simulink model "pure_pursuit"  (R2025b)
settings: Solver=ode45  StartTime=0.0  StopTime=inf  RelTol=1e-3
model workspace (MAT data in the model file):
  SL_ROS_VariableLengthArrays_MaxSizes.CommonInfo.ArrayTruncateAction = 'EmitWarning'
  SL_ROS_VariableLengthArrays_MaxSizes.MsgTypeMap = containers.Map
  SL_ROS_VariableLengthArrays_MaxSizes.MsgTypeMap.serialization.keys = {'autoware_planning_msgs/Path'}
  SL_ROS_VariableLengthArrays_MaxSizes.MsgTypeMap.serialization.values{1}(1).PropertyName = 'left_bound'
  SL_ROS_VariableLengthArrays_MaxSizes.MsgTypeMap.serialization.values{1}(1).DataType = 'geometry_msgs/Point'
  SL_ROS_VariableLengthArrays_MaxSizes.MsgTypeMap.serialization.values{1}(1).MaxLength = 159
  SL_ROS_VariableLengthArrays_MaxSizes.MsgTypeMap.serialization.values{1}(2).PropertyName = 'points'
  SL_ROS_VariableLengthArrays_MaxSizes.MsgTypeMap.serialization.values{1}(2).DataType = 'autoware_planning_msgs/PathPoint'
  SL_ROS_VariableLengthArrays_MaxSizes.MsgTypeMap.serialization.values{1}(2).MaxLength = 159
  SL_ROS_VariableLengthArrays_MaxSizes.MsgTypeMap.serialization.values{1}(3).PropertyName = 'right_bound'
  SL_ROS_VariableLengthArrays_MaxSizes.MsgTypeMap.serialization.values{1}(3).DataType = 'geometry_msgs/Point'
  SL_ROS_VariableLengthArrays_MaxSizes.MsgTypeMap.serialization.values{1}(3).MaxLength = 159
  SL_ROS_VariableLengthArrays_MaxSizes.MsgTypeMap.serialization.uniformity = 0
  SL_ROS_VariableLengthArrays_MaxSizes.MsgTypeMap.serialization.keyType = 'char'
  SL_ROS_VariableLengthArrays_MaxSizes.MsgTypeMap.serialization.valueType = 'any'
values from neighbouring files (symbols this model uses):
  L = 3    [autoware_referance_path_creater.m]    (also in pure_pursuit_parameters.m)
  ld = 5    [autoware_referance_path_creater.m]    (also in pure_pursuit_parameters.m = 3)
  max_ld = 10    [autoware_referance_path_creater.m]    (also in pure_pursuit_parameters.m)
  max_steer_cmd = 0.5    [autoware_referance_path_creater.m]    (also in pure_pursuit_parameters.m)
  max_vel = 10    [autoware_referance_path_creater.m]    (also in pure_pursuit_parameters.m)
  min_ld = 3    [autoware_referance_path_creater.m]    (also in pure_pursuit_parameters.m)
  min_steer_cmd = 0.0    (= 0)    [autoware_referance_path_creater.m]    (also in pure_pursuit_parameters.m)
  min_vel = 5    [autoware_referance_path_creater.m]    (also in pure_pursuit_parameters.m)
  psi_o = atan2(dy0, dx0)    [autoware_referance_path_creater.m]    (also in pure_pursuit_parameters.m = 0)
  x_mean = x_mean(:)    [load_onnx_params.m]    (also in scaler_params.mat = [28.1934460749 74.6575043237 -0.0407059238974])
  X_o = refPose(1,1)    [autoware_referance_path_creater.m]    (also in pure_pursuit_parameters.m)
  x_std = x_std(:)    [load_onnx_params.m]    (also in scaler_params.mat = [17.0789640418 18.417349091 0.180735882078])
  xRef = refPose(:,1)    [autoware_referance_path_creater.m]    (also in pure_pursuit_parameters.m)
  y_mean = y_mean(:)    [load_onnx_params.m]    (also in scaler_params.mat = [7.96333555037 8.54523967985])
  Y_o = refPose(1,2)    [autoware_referance_path_creater.m]    (also in pure_pursuit_parameters.m)
  y_std = y_std(:)    [load_onnx_params.m]    (also in scaler_params.mat = [1.60598708046 1.14713361971])
  yRef = refPose(:,2)    [autoware_referance_path_creater.m]    (also in pure_pursuit_parameters.m)
libraries: autolibshared x6, robotalgslib x5, robotmobilelib x2, pycoexlib x1, ros2lib x1
settings Model: Creator=omer  LastModifiedBy=omer
settings OptimizationCC: DefaultParameterBehavior=Inlined  EnhancedBackFolding=on  PassReuseOutputArgsAs=Individual arguments  ZeroExternalMemoryAtStartup=off  ZeroInternalMemoryAtStartup=off  MaxStackSize=64  OptimizeBlockOrder=speed  DifferentSizesBufferReuse=on  OptimizationCustomize=off  EfficientTunableParamExpr=on
settings DebuggingCC: AlgebraicLoopMsg=none  ParameterTunabilityLossMsg=error
settings HardwareCC: ProdBitPerLong=64.0  ProdHWDeviceType=Intel->x86-64 (Linux 64)
settings SFSimCC: MATLABDynamicMemAlloc=off
settings RTWCC: SystemTargetFile=ert.tlc  HardwareBoard=Robot Operating System 2 (ROS 2)  TLCOptions="-aInlineSetEventsForThisBaseRateFcn=TLC_FALSE -aSuppressMultiTaskScheduler=TLC_FALSE  -aRateBasedStepFcn=0"  TemplateMakefile=ert_default_tmf  Toolchain=Colcon Tools  TargetLang=C++  Description=Embedded Coder
settings CodeAppCC: ForceParamTrailComments=on  IgnoreCustomStorageClasses=off  OperatorAnnotations=on  SimulinkDataObjDesc=on  SFDataObjDesc=on  InsertBlockDesc=on
settings ERTTargetCC: ExtModeTransport=2.0  ExtModeStaticAlloc=on  ExtModeAutomaticAllocSize=off  ExtModeMexFile=ext_xcp  ExtModeIntrfLevel=Level2 - Open  RootIOFormat=Structure reference  CodeInterfacePackaging=C++ class

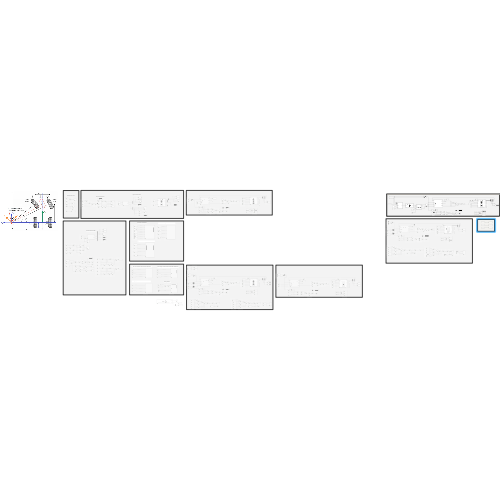
[thumbnail: Simulink's stored preview of the top-level diagram]
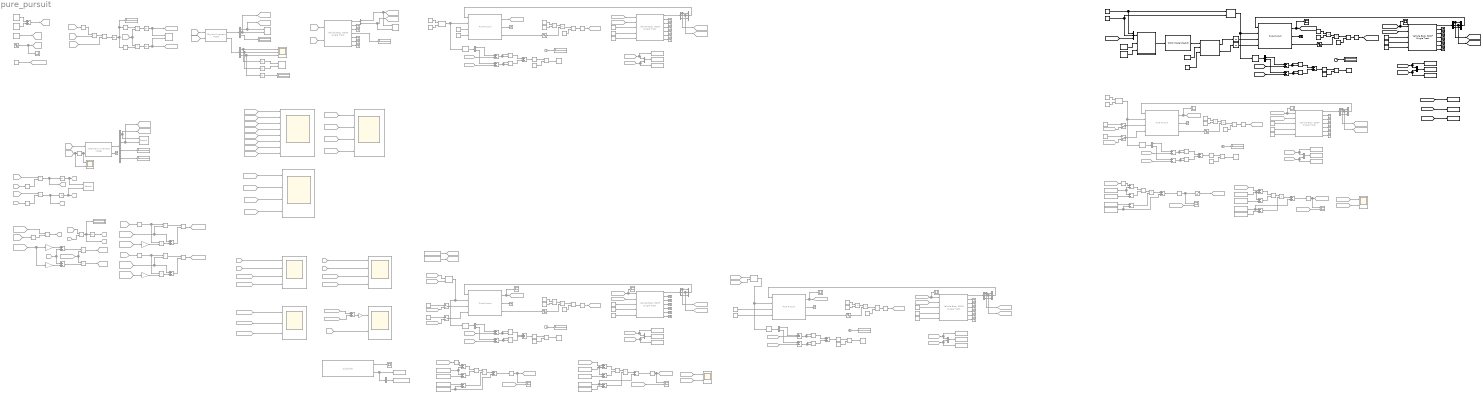
== system pure_pursuit ==
  note: Bicycle Kinematics Model
  note: Bicycle Kinematics Model
  note: Ackerman Kinematics Model
  note: Kinematics Model Inputs
  note: All Kinematics Model Results
  note: Built in and custom Bicycle Kinematics Model Results
  note: Bicycle and Ackerman Kinematics Model Results
  note: Built-in and custom Ackermann Kinematics Model Results
  note: Custom Bicycle and custom Ackermann Kinematics Model Results
  note: Velocity Calculation
  note: Steering Angle Calculation
  Abs{,1..5} (6 alike) : Abs  Commented=on  SaturateOnIntegerOverflow=off
  Ackermann Kinematic Model : robotmobilelib/Ackermann Kinematic Model  Commented=on  WheelBase=3  VehicleSpeedRange=[-10 10]  MaxSteeringAngle=pi/4  InitialState=[0; 0; 0; 0]  SimulateUsing=Interpreted execution
  Add{,1..5,8,11,19,23,32,34} (12 alike) : Sum  Commented=on
  Add{6..7,9..10,12,15..16,22,24,27..28,33,35..36} (14 alike) : Sum  Commented=on  Inputs=+-
  Add{13..14,17..18,25..26,29,31} (8 alike) : Sum  Commented=on  Inputs=-+
  Add37 : Sum  Inputs=+-
  Add38 : Sum
  Add39 : Sum  Inputs=+-
  Angular Velocity : Sin  Commented=on  Amplitude=0.6  Frequency=0.2  SampleTime=0
  Atan{,1,3..4} (4 alike) : Trigonometry  Commented=on  Operator=atan
  Atan5 : Trigonometry  Operator=atan
  Bicycle Kinematic Model : robotmobilelib/Bicycle Kinematic Model  Commented=on  VehicleInputs=Vehicle Speed & Steering Angle  WheelBase=3  VehicleSpeedRange=[-10 10]  MaxSteeringAngle=pi/4  InitialState=[0; 0; 0]  SimulateUsing=Interpreted execution
  Bus Selector{,2,5..6} (4 alike) : BusSelector  Commented=on  OutputSignals=InertFrm.Cg.Disp.X,InertFrm.Cg.Disp.Y,InertFrm.Cg.Ang.psi
  Bus Selector1 : BusSelector  Commented=on  OutputSignals=InertFrm.Cg.Disp.X,InertFrm.Cg.Disp.Y
  Bus Selector4 : BusSelector  Commented=on  OutputSignals=points
  Bus Selector7 : BusSelector  OutputSignals=InertFrm.Cg.Disp.X,InertFrm.Cg.Disp.Y,InertFrm.Cg.Ang.psi
  Clock{,1,3..4} (4 alike) : Clock  Commented=on
  Clock5 : Clock
  Constant : Constant  Commented=on  Value=2.5
  Constant{1,10,42,57} (4 alike) : Constant  Commented=on  Value=2
  Constant{8,11,13,21,43,51,58,70} (8 alike) : Constant  Commented=on  Value=ld
  Constant12 : Constant  Commented=on
  Constant14 : Constant  Commented=on  Value=0.5
  Constant{2,15,45,64} (4 alike) : Constant  Commented=on  Value=X_o
  Constant{3,16,46,65} (4 alike) : Constant  Commented=on  Value=Y_o
  Constant{4,17,47,66} (4 alike) : Constant  Commented=on  Value=psi_o
  Constant18 : Constant  Commented=on  Value=xRef
  Constant19 : Constant  Commented=on  Value=yRef
  Constant20 : Constant  Commented=on  Value=10
  Constant{9,22,52,71} (4 alike) : Constant  Commented=on  Value=L
  Constant23 : Constant  Commented=on  Value=min_steer_cmd
  Constant24 : Constant  Commented=on  Value=max_steer_cmd
  Constant{25,29,55,59} (4 alike) : Constant  Commented=on  Value=min_ld
  Constant{26,30,56,60} (4 alike) : Constant  Commented=on  Value=max_ld
  Constant31 : Constant  Commented=on  Value=min_vel
  Constant32 : Constant  Commented=on  Value=max_vel
  Constant44 : Constant  Commented=on
  Constant48 : Constant  Commented=on  Value=xRef
  Constant49 : Constant  Commented=on  Value=yRef
  Constant5 : Constant  Commented=on  Value=xRef
  Constant50 : Constant  Commented=on  Value=5
  Constant53 : Constant  Commented=on  Value=min_steer_cmd
  Constant54 : Constant  Commented=on  Value=max_steer_cmd
  Constant6 : Constant  Commented=on  Value=yRef
  Constant61 : Constant  Commented=on  Value=min_vel
  Constant62 : Constant  Commented=on  Value=max_vel
  Constant63 : Constant  Commented=on
  Constant67 : Constant  Value=2
  Constant68 : Constant  Value=ld
  Constant69 : Constant  Commented=on  Value=10
  Constant7 : Constant  Commented=on  Value=10
  Constant72 : Constant  Value=0.5
  Constant73 : Constant  Value=X_o
  Constant74 : Constant  Value=Y_o
  Constant75 : Constant  Value=psi_o
  Constant76 : Constant  Value=xRef
  Constant77 : Constant  Value=yRef
  Constant78 : Constant  Value=x_mean
  Constant79 : Constant  Value=x_std
  Constant80 : Constant  Value=L
  Constant81 : Constant  Value=y_mean
  Constant82 : Constant  Value=y_std
  Cos : Trigonometry  Commented=on  Operator=cos
  Cos1 : Trigonometry  Commented=on  Operator=cos
  Cos2 : Trigonometry  Commented=on
  Demux : Demux  Commented=on  Outputs=3
  Demux1 : Demux  Commented=on  Outputs=3
  Demux2 : Demux  Commented=on
  Demux{3..4,6..7} (4 alike) : Demux  Commented=on  Outputs=2
  Demux8 : Demux  Outputs=2
  Derivative : Derivative  Commented=on
  Display{,1..8,10..11} (11 alike) : Display  Commented=on
  Display12 : Display
  Divide{,1..8,10..13} (13 alike) : Product  Commented=on  Inputs=*/
  Divide14 : Product  Inputs=*/
  Dot Product{,1..3,6..9} (8 alike) : DotProduct  Commented=on  OutDataTypeStr=Inherit: Inherit via internal rule
  Dot Product10 : DotProduct  OutDataTypeStr=Inherit: Inherit via internal rule
  Dot Product11 : DotProduct  OutDataTypeStr=Inherit: Inherit via internal rule
  From{,2,5,7..8,37,43,45,56} (9 alike) : From  Commented=on  GotoTag=LinVel
  From{1,3,6,9,38,48,51,57} (8 alike) : From  Commented=on  GotoTag=SteerAngle
  From10 : From  Commented=on  GotoTag=bicycle_block_x
  From11 : From  Commented=on  GotoTag=bicycle_block_y
  From12 : From  Commented=on  GotoTag=bicycle_sub_x
  From13 : From  Commented=on  GotoTag=bicycle_sub_y
  From14 : From  Commented=on  GotoTag=ackerman_block_x
  From15 : From  Commented=on  GotoTag=ackerman_block_y
  From16 : From  Commented=on  GotoTag=bicycle_vel_x
  From17 : From  Commented=on  GotoTag=bicycle_vel_y
  From18 : From  Commented=on  GotoTag=bicycle_block_x
  From19 : From  Commented=on  GotoTag=bicycle_block_y
  From20 : From  Commented=on  GotoTag=bicycle_sub_x
  From21 : From  Commented=on  GotoTag=bicycle_sub_y
  From22 : From  Commented=on  GotoTag=bicycle_block_x
  From23 : From  Commented=on  GotoTag=bicycle_block_y
  From24 : From  Commented=on  GotoTag=ackerman_block_x
  From25 : From  Commented=on  GotoTag=ackerman_block_y
  From26 : From  Commented=on  GotoTag=x
  From27 : From  Commented=on  GotoTag=x_feedback
  From28 : From  Commented=on  GotoTag=y_feedback
  From29 : From  Commented=on  GotoTag=calculated_lin_vel
  From30 : From  Commented=on  GotoTag=y
  From31 : From  Commented=on  GotoTag=ackerman_block_x
  From32 : From  Commented=on  GotoTag=ackerman_block_y
  From33 : From  Commented=on  GotoTag=x
  From34 : From  Commented=on  GotoTag=y
  From35 : From  Commented=on  GotoTag=bicycle_sub_x
  From36 : From  Commented=on  GotoTag=bicycle_sub_y
  From{4,39,49,52} (4 alike) : From  Commented=on  GotoTag=WheelBase
  From40 : From  Commented=on  GotoTag=WheelSeparation
  From41 : From  Commented=on  GotoTag=R
  From42 : From  Commented=on  GotoTag=R
  From44 : From  Commented=on  GotoTag=q
  From46 : From  Commented=on  GotoTag=q
  From47 : From  Commented=on  GotoTag=q_dot
  From50 : From  Commented=on  GotoTag=WheelSeparation
  From53 : From  Commented=on  GotoTag=WheelSeparation
  From54 : From  Commented=on  GotoTag=v_inner_wheel
  From55 : From  Commented=on  GotoTag=v_outer_wheel
  From58 : From  Commented=on  GotoTag=InnerSteeringAngle
  From59 : From  Commented=on  GotoTag=OutterSteeringAngle
  From{60,64..65,69..70,80..81,85..86} (9 alike) : From  Commented=on  GotoTag=steering_cmd
  From61 : From  Commented=on  GotoTag=x_feedback
  From62 : From  Commented=on  GotoTag=y_feedback
  From63 : From  Commented=on  GotoTag=calculated_lin_vel
  From{66..67,77,82..83,91} (6 alike) : From  Commented=on  GotoTag=regulated_ld
  From{68,78,84,92} (4 alike) : From  Commented=on  GotoTag=regulated_vel
  From75 : From  Commented=on  GotoTag=x_feedback
  From76 : From  Commented=on  GotoTag=y_feedback
  From79 : From  Commented=on  GotoTag=calculated_lin_vel
  From87 : From  Commented=on  GotoTag=x_feedback2
  From88 : From  Commented=on  GotoTag=y_feedback2
  From89 : From  Commented=on  GotoTag=calculated_lin_vel2
  From90 : From  Commented=on  GotoTag=steering_cmd2
  From93 : From  Commented=on  GotoTag=test_path_x
  From94 : From  Commented=on  GotoTag=test_path_y
  From95 : From  Commented=on  GotoTag=test_path_x
  From96 : From  Commented=on  GotoTag=test_path_y
  Gain : Gain  Commented=on  Gain=-0.5
  Gain1 : Gain  Commented=on  Gain=0.5
  Gain2 : Gain  Commented=on  Gain=-0.5
  Gain3 : Gain  Commented=on  Gain=0.5
  Gain4 : Gain  Commented=on  Gain=0.5
  Goto : Goto  Commented=on  GotoTag=LinVel
  Goto1 : Goto  Commented=on  GotoTag=SteerAngle
  Goto10 : Goto  Commented=on  GotoTag=bicycle_vel_y
  Goto11 : Goto  Commented=on  GotoTag=WheelSeparation
  Goto12 : Goto  Commented=on  GotoTag=calculated_lin_vel
  Goto13 : Goto  Commented=on  GotoTag=steering_cmd
  Goto14 : Goto  Commented=on  GotoTag=x
  Goto15 : Goto  Commented=on  GotoTag=y
  Goto16 : Goto  Commented=on  GotoTag=R
  Goto17 : Goto  Commented=on  GotoTag=q_dot
  Goto18 : Goto  Commented=on  GotoTag=v_inner_wheel
  Goto19 : Goto  Commented=on  GotoTag=v_outer_wheel
  Goto2 : Goto  Commented=on  GotoTag=bicycle_sub_x
  Goto20 : Goto  Commented=on  GotoTag=x_dot
  Goto21 : Goto  Commented=on  GotoTag=y_dot
  Goto22 : Goto  Commented=on  GotoTag=InnerSteeringAngle
  Goto23 : Goto  Commented=on  GotoTag=OutterSteeringAngle
  Goto24 : Goto  Commented=on  GotoTag=q
  Goto25 : Goto  Commented=on  GotoTag=x_feedback
  Goto26 : Goto  Commented=on  GotoTag=y_feedback
  Goto27 : Goto  Commented=on  GotoTag=calculated_lin_vel
  Goto28 : Goto  Commented=on  GotoTag=steering_cmd
  Goto29 : Goto  Commented=on  GotoTag=x_feedback
  Goto3 : Goto  Commented=on  GotoTag=WheelBase
  Goto30 : Goto  Commented=on  GotoTag=y_feedback
  Goto31 : Goto  Commented=on  GotoTag=regulated_ld
  Goto32 : Goto  Commented=on  GotoTag=regulated_vel
  Goto37 : Goto  Commented=on  GotoTag=calculated_lin_vel
  Goto38 : Goto  Commented=on  GotoTag=steering_cmd
  Goto39 : Goto  Commented=on  GotoTag=x_feedback
  Goto4 : Goto  Commented=on  GotoTag=bicycle_sub_y
  Goto40 : Goto  Commented=on  GotoTag=y_feedback
  Goto41 : Goto  Commented=on  GotoTag=regulated_ld
  Goto42 : Goto  Commented=on  GotoTag=regulated_vel
  Goto43 : Goto  Commented=on  GotoTag=calculated_lin_vel2
  Goto44 : Goto  Commented=on  GotoTag=steering_cmd2
  Goto45 : Goto  Commented=on  GotoTag=x_feedback2
  Goto46 : Goto  Commented=on  GotoTag=y_feedback2
  Goto47 : Goto  Commented=on  GotoTag=test_path_x
  Goto48 : Goto  Commented=on  GotoTag=test_path_y
  Goto5 : Goto  Commented=on  GotoTag=bicycle_block_x
  Goto6 : Goto  Commented=on  GotoTag=bicycle_block_y
  Goto7 : Goto  Commented=on  GotoTag=ackerman_block_x
  Goto8 : Goto  Commented=on  GotoTag=ackerman_block_y
  Goto9 : Goto  Commented=on  GotoTag=bicycle_vel_x
  Integrator{,1..5,8,10..11} (9 alike) : Integrator  Commented=on
  Less Than{,1,3..4} (4 alike) : RelationalOperator  Commented=on  Operator=<  OutDataTypeStr=boolean  RndMeth=Simplest  InputSameDT=off
  Less Than5 : RelationalOperator  Operator=<  OutDataTypeStr=boolean  RndMeth=Simplest  InputSameDT=off
  Linear Velocity : Constant  Commented=on
  MATLAB Function : MATLAB Function  TreatAsAtomicUnit=on
  MATLAB Function1 : MATLAB Function  TreatAsAtomicUnit=on
  Manual Switch : ManualSwitch  Commented=on  CurrentSetting=0
  Manual Switch1 : ManualSwitch  Commented=on  CurrentSetting=0
  Manual Switch2 : ManualSwitch  Commented=on
  Manual Switch3 : ManualSwitch  Commented=on
  Matrix Concatenate{,1,3..4} (4 alike) : Concatenate  Commented=on  Mode=Multidimensional array  ConcatenateDimension=2
  Matrix Concatenate5 : Concatenate  Mode=Multidimensional array  ConcatenateDimension=2
  Mux{,2,6,8} (4 alike) : Mux  Commented=on  Inputs=3
  Mux{1,3,7,9} (4 alike) : Mux  Commented=on  Inputs=2
  Mux10 : Mux  Inputs=3
  Mux11 : Mux  Inputs=2
  ONNX Model Predict : pycoexlib/ONNX Model Predict  ModelFile=/home/omer/custom_pure_pursuit/simulink_models/lookahead_velocity_model.onnx  ExecutionProviders=AzureExecutionProvider, CPUExecutionProvider  InputTable={ 'input', 'float32', '', '2' }  OutputTable={ 'output', '', '2' }  SampleTime=0.1  InputDatatypes=float32  InputNumDims=2  InputPermutations=[]  OutputPermutations=[]  PythonCoexecutionBlockType=ONNXModelBlock  VariableOutputMaxSizes=2
  Product{,1..16,19..24} (23 alike) : Product  Commented=on
  Product25 : Product
  Product26 : Product
  Pure Pursuit{,1,3..4} (4 alike) : robotalgslib/Pure Pursuit  Commented=on  DesiredLinearVelocityPort=on  DesiredLinearVelocity=0.1  MaxAngularVelocity=1.0  LookaheadDistancePort=on  LookaheadDistance=1.0  TargetDirPort=on  SimulateUsing=Code generation
      settings: LibrarySourceBlock=navlib/Control Algorithms/Pure Pursuit
  Pure Pursuit5 : robotalgslib/Pure Pursuit  DesiredLinearVelocityPort=on  DesiredLinearVelocity=0.1  MaxAngularVelocity=1.0  LookaheadDistancePort=on  LookaheadDistance=1.0  TargetDirPort=on  SimulateUsing=Code generation
      settings: LibrarySourceBlock=navlib/Control Algorithms/Pure Pursuit
  Saturation : Saturate  Commented=on  UpperLimit=10  LowerLimit=0.1
  Scope : Scope  Commented=on  NumInputPorts=3
      settings: ActiveDisplayYMinimum=-1  ActiveDisplayYMaximum=1
  Scope1 : Scope  Commented=on  NumInputPorts=8
      settings: ActiveDisplayYMinimum=-455.06067529174624  ActiveDisplayYMaximum=417.5791885173104
  Scope{3,10,13,17,20..23} (8 alike) : Scope  Commented=on
      Scope10 settings: ActiveDisplayYMinimum=-2.1920698371442371  ActiveDisplayYMaximum=1.9657865216785007  DataLoggingVariableName=ScopeData10
      Scope13 settings: ActiveDisplayYMinimum=2.3400699446242892  ActiveDisplayYMaximum=6.7058191213881608  DataLoggingVariableName=ScopeData13
      Scope17 settings: ActiveDisplayYMinimum=-6.54243807856459  ActiveDisplayYMaximum=6.3199793503646529  DataLoggingVariableName=ScopeData17
      Scope20 settings: ActiveDisplayYMinimum=2.3400699446242892  ActiveDisplayYMaximum=6.7058191213881608  DataLoggingVariableName=ScopeData20
      Scope21 settings: ActiveDisplayYMinimum=2.3400699446242892  ActiveDisplayYMaximum=6.7058191213881608  DataLoggingVariableName=ScopeData21
      Scope22 settings: ActiveDisplayYMinimum=-6.54243807856459  ActiveDisplayYMaximum=6.3199793503646529  DataLoggingVariableName=ScopeData22
      Scope23 settings: ActiveDisplayYMinimum=-6.54243807856459  ActiveDisplayYMaximum=6.3199793503646529  DataLoggingVariableName=ScopeData23
      Scope3 settings: ActiveDisplayYMinimum=-1.3341695524882851  ActiveDisplayYMaximum=1.7529271348584103  DataLoggingVariableName=ScopeData3
  Scope{7,9,11..12,14..15,19,24} (8 alike) : Scope  Commented=on  NumInputPorts=2
      Scope11 settings: ActiveDisplayYMinimum=-16.400538939289639  ActiveDisplayYMaximum=34.683500692121072  DataLoggingVariableName=ScopeData11
      Scope12 settings: ActiveDisplayYMinimum=0.60593319304369331  ActiveDisplayYMaximum=15.551193421535297  DataLoggingVariableName=ScopeData12
      Scope14 settings: ActiveDisplayYMinimum=-82.294699623194319  ActiveDisplayYMaximum=306.26602380301892  DataLoggingVariableName=ScopeData14
      Scope15 settings: ActiveDisplayYMinimum=-10.847724246816968  ActiveDisplayYMaximum=9.18035383339083  DataLoggingVariableName=ScopeData15
      Scope19 settings: ActiveDisplayYMinimum=-81.236983986469738  ActiveDisplayYMaximum=268.25133590848907  DataLoggingVariableName=ScopeData19
      Scope24 settings: ActiveDisplayYMinimum=-22.851027240799276  ActiveDisplayYMaximum=28.83992030131644  DataLoggingVariableName=ScopeData24
      Scope7 settings: ActiveDisplayYMinimum=-3.4268970997372428  ActiveDisplayYMaximum=28.386536930736913  DataLoggingVariableName=ScopeData7
      Scope9 settings: ActiveDisplayYMinimum=-1.3341695524882851  ActiveDisplayYMaximum=1.7529271348584103  DataLoggingVariableName=ScopeData9
  Scope{2,4..6} (4 alike) : Scope  Commented=on  NumInputPorts=4
      Scope2 settings: ActiveDisplayYMinimum=0.32572897203293749  ActiveDisplayYMaximum=21.907338374210166  DataLoggingVariableName=ScopeData2
      Scope4 settings: ActiveDisplayYMinimum=32.57770845291958  ActiveDisplayYMaximum=624.63304863060557  DataLoggingVariableName=ScopeData4
      Scope5 settings: ActiveDisplayYMinimum=-4.3902728806219606  ActiveDisplayYMaximum=29.013832851375891  DataLoggingVariableName=ScopeData5
      Scope6 settings: ActiveDisplayYMinimum=-3.4268970997372428  ActiveDisplayYMaximum=28.386536930736913  DataLoggingVariableName=ScopeData6
  Scope25 : Scope
      settings: ActiveDisplayYMinimum=2.3400699446242892  ActiveDisplayYMaximum=6.7058191213881608  DataLoggingVariableName=ScopeData25
  Scope26 : Scope
      settings: ActiveDisplayYMinimum=-6.54243807856459  ActiveDisplayYMaximum=6.3199793503646529  DataLoggingVariableName=ScopeData26
  Scope8 : Scope  Commented=on  NumInputPorts=3
      settings: ActiveDisplayYMinimum=-4.3617646340530536  ActiveDisplayYMaximum=11.80186087051403  DataLoggingVariableName=ScopeData8
  Selector{,1,3..4} (4 alike) : Selector  Commented=on  NumberOfDimensions=2  InputPortWidth=3  IndexOptions=Index vector (dialog),Index vector (dialog)  Indices=48,[1:2]  OutputSizes=1,1
  Selector5 : Selector  NumberOfDimensions=2  InputPortWidth=3  IndexOptions=Index vector (dialog),Index vector (dialog)  Indices=48,[1:2]  OutputSizes=1,1
  Sin : Trigonometry  Commented=on
  Sine Wave{,1,3..4} (4 alike) : Sin  Commented=on  TimeSource=Use external signal  SampleTime=0
  Sine Wave5 : Sin  TimeSource=Use external signal  SampleTime=0
  Square{,1,3..4} (4 alike) : Math  Commented=on  Operator=square
  Square5 : Math  Operator=square
  Stop Simulation{,1,3..4} (4 alike) : Stop  Commented=on
  Stop Simulation5 : Stop
  Subscribe : ros2lib/Subscribe  Commented=on  topicSource=Select from ROS network  topic=/planning/scenario_planning/lane_driving/behavior_planning/path  messageType=autoware_planning_msgs/Path  sampleTime=-1  QOSHistory=Keep last  QOSDepth=10  QOSReliability=Reliable  QOSDurability=Volatile  QOSDeadline=Inf  QOSLifespan=Inf  QOSLiveliness=Automatic  QOSLeaseDuration=Inf  QOSAvoidROSNamespaceConventions=off
  Tan{,2..4} (4 alike) : Trigonometry  Commented=on  Operator=tan
  Terminator{1..20,28..41} (34 alike) : Terminator  Commented=on
  Terminator{42..48} (7 alike) : Terminator
  To Workspace : ToWorkspace  Commented=on  VariableName=tracked_path  SampleTime=-1
      settings: Save2DSignal=2-D array (concatenate along first dimension)
  To Workspace1 : ToWorkspace  Commented=on  VariableName=tracked_path_x  SampleTime=-1
      settings: Save2DSignal=2-D array (concatenate along first dimension)
  To Workspace10 : ToWorkspace  Commented=on  VariableName=autoware_path_array  SaveFormat=Timeseries  SampleTime=-1
      settings: Save2DSignal=2-D array (concatenate along first dimension)
  To Workspace11 : ToWorkspace  Commented=on  VariableName=tracked_path  SampleTime=-1
      settings: Save2DSignal=2-D array (concatenate along first dimension)
  To Workspace12 : ToWorkspace  Commented=on  VariableName=tracked_path_x  SampleTime=-1
      settings: Save2DSignal=2-D array (concatenate along first dimension)
  To Workspace13 : ToWorkspace  Commented=on  VariableName=tracked_path_y  SampleTime=-1
      settings: Save2DSignal=2-D array (concatenate along first dimension)
  To Workspace14 : ToWorkspace  Commented=on  VariableName=tracked_path2  SampleTime=-1
      settings: Save2DSignal=2-D array (concatenate along first dimension)
  To Workspace15 : ToWorkspace  Commented=on  VariableName=tracked_path_x2  SampleTime=-1
      settings: Save2DSignal=2-D array (concatenate along first dimension)
  To Workspace16 : ToWorkspace  Commented=on  VariableName=tracked_path_y2  SampleTime=-1
      settings: Save2DSignal=2-D array (concatenate along first dimension)
  To Workspace17 : ToWorkspace  VariableName=steering_ref  SampleTime=-1
      settings: Save2DSignal=2-D array (concatenate along first dimension)
  To Workspace18 : ToWorkspace  VariableName=velocity_ref  SampleTime=-1
      settings: Save2DSignal=2-D array (concatenate along first dimension)
  To Workspace19 : ToWorkspace  VariableName=look_ahead_ref  SampleTime=-1
      settings: Save2DSignal=2-D array (concatenate along first dimension)
  To Workspace2 : ToWorkspace  Commented=on  VariableName=tracked_path_y  SampleTime=-1
      settings: Save2DSignal=2-D array (concatenate along first dimension)
  To Workspace20 : ToWorkspace  VariableName=tracked_path_nn  SampleTime=-1
      settings: Save2DSignal=2-D array (concatenate along first dimension)
  To Workspace21 : ToWorkspace  VariableName=tracked_path_x_nn  SampleTime=-1
      settings: Save2DSignal=2-D array (concatenate along first dimension)
  To Workspace22 : ToWorkspace  VariableName=tracked_path_y_nn  SampleTime=-1
      settings: Save2DSignal=2-D array (concatenate along first dimension)
  To Workspace3 : ToWorkspace  Commented=on  VariableName=autoware_path  SaveFormat=Timeseries  SampleTime=-1
  To Workspace4 : ToWorkspace  Commented=on  VariableName=tracked_path  SampleTime=-1
      settings: Save2DSignal=2-D array (concatenate along first dimension)
  To Workspace5 : ToWorkspace  Commented=on  VariableName=tracked_path_x  SampleTime=-1
      settings: Save2DSignal=2-D array (concatenate along first dimension)
  To Workspace6 : ToWorkspace  Commented=on  VariableName=tracked_path_y  SampleTime=-1
      settings: Save2DSignal=2-D array (concatenate along first dimension)
  Unit Delay : UnitDelay  InitialCondition=5  SampleTime=0.1  HasFrameUpgradeWarning=on
  Unit Delay1 : UnitDelay  InitialCondition=5  SampleTime=0.1  HasFrameUpgradeWarning=on
  Vector Concatenate : Concatenate  NumInputs=3
  Vehicle Body 3DOF Single Track{,2,4..5} (4 alike) : autolibshared/Vehicle Body 3DOF Single Track  Commented=on  trackMode=Single (bicycle)  inputMode=External longitudinal velocity  frontSteerMode=on  rearSteerMode=off  windMode=off  muMode=off  extFMode=off  extMMode=off  htchFMode=off  htchMMode=off  extXo=on  extpsio=on  extxdoto=off  extro=off  extYo=on  extTamb=off  extydoto=off  aMode=2  NF=2  NR=2  m=2000  a=1.4  b=1.6  h=0.35  dh=1  hh=0.2  X_o=0  xdot_o=0  CalphaMode=off  sigmaMode=on  d=0  hl=0  w=[1.4,1.4]  Cy_f=12e3  Cy_r=11e3  sigma_f=.1  sigma_r=.1  alpha_f_brk=[-0.785, -0.628, -0.471, -0.314, -0.157, 0.000, 0.157, 0.314, 0.471, 0.628, 0.785]  Cy_f_data=[2000, 3000, 4000, 5500, 7000, 9000, 7000, 5500, 4000, 3000, 2000]  alpha_r_brk=[-0.785, -0.628, -0.471, -0.314, -0.157, 0.000, 0.157, 0.314, 0.471, 0.628, 0.785]  Cy_r_data=[2000, 3000, 4000, 5500, 7000, 9000, 7000, 5500, 4000, 3000, 2000]  Y_o=0  ydot_o=0  Izz=4000  psi_o=0  r_o=0  Af=2  Cd=.3  Cl=.1  Cpm=.1  beta_w=[0 0.01:0.01:0.3]  Cs=[0:0.03:0.9]  Cym=[0 1e-6:0.01:0.3]  Pabs=101325  Tair=273  g=9.81  mu=1  xdot_tol=.01  Fznom=5000  Fxtire_sat=7e4  Fytire_sat=7e4  longOff=0  latOff=0  vertOff=0  wrapAng=off
      settings: LibrarySourceBlock=vehdynlibeom/Vehicle Body 3DOF Dual Track
  Vehicle Body 3DOF Single Track1 : autolibshared/Vehicle Body 3DOF Single Track  Commented=on  trackMode=Single (bicycle)  inputMode=External longitudinal velocity  frontSteerMode=on  rearSteerMode=off  windMode=off  muMode=off  extFMode=off  extMMode=off  htchFMode=off  htchMMode=off  extXo=off  extpsio=off  extxdoto=off  extro=off  extYo=off  extTamb=off  extydoto=off  aMode=2  NF=2  NR=2  m=2000  a=1.4  b=1.6  h=0.35  dh=1  hh=0.2  X_o=0  xdot_o=0  CalphaMode=off  sigmaMode=on  d=0  hl=0  w=[1.4,1.4]  Cy_f=12e3  Cy_r=11e3  sigma_f=.1  sigma_r=.1  alpha_f_brk=[-0.785, -0.628, -0.471, -0.314, -0.157, 0.000, 0.157, 0.314, 0.471, 0.628, 0.785]  Cy_f_data=[2000, 3000, 4000, 5500, 7000, 9000, 7000, 5500, 4000, 3000, 2000]  alpha_r_brk=[-0.785, -0.628, -0.471, -0.314, -0.157, 0.000, 0.157, 0.314, 0.471, 0.628, 0.785]  Cy_r_data=[2000, 3000, 4000, 5500, 7000, 9000, 7000, 5500, 4000, 3000, 2000]  Y_o=0  ydot_o=0  Izz=4000  psi_o=0  r_o=0  Af=2  Cd=.3  Cl=.1  Cpm=.1  beta_w=[0 0.01:0.01:0.3]  Cs=[0:0.03:0.9]  Cym=[0 1e-6:0.01:0.3]  Pabs=101325  Tair=273  g=9.81  mu=1  xdot_tol=.01  Fznom=5000  Fxtire_sat=7e4  Fytire_sat=7e4  longOff=0  latOff=0  vertOff=0  wrapAng=off
      settings: LibrarySourceBlock=vehdynlibeom/Vehicle Body 3DOF Dual Track
  Vehicle Body 3DOF Single Track6 : autolibshared/Vehicle Body 3DOF Single Track  trackMode=Single (bicycle)  inputMode=External longitudinal velocity  frontSteerMode=on  rearSteerMode=off  windMode=off  muMode=off  extFMode=off  extMMode=off  htchFMode=off  htchMMode=off  extXo=on  extpsio=on  extxdoto=off  extro=off  extYo=on  extTamb=off  extydoto=off  aMode=2  NF=2  NR=2  m=2000  a=1.4  b=1.6  h=0.35  dh=1  hh=0.2  X_o=0  xdot_o=0  CalphaMode=off  sigmaMode=on  d=0  hl=0  w=[1.4,1.4]  Cy_f=12e3  Cy_r=11e3  sigma_f=.1  sigma_r=.1  alpha_f_brk=[-0.785, -0.628, -0.471, -0.314, -0.157, 0.000, 0.157, 0.314, 0.471, 0.628, 0.785]  Cy_f_data=[2000, 3000, 4000, 5500, 7000, 9000, 7000, 5500, 4000, 3000, 2000]  alpha_r_brk=[-0.785, -0.628, -0.471, -0.314, -0.157, 0.000, 0.157, 0.314, 0.471, 0.628, 0.785]  Cy_r_data=[2000, 3000, 4000, 5500, 7000, 9000, 7000, 5500, 4000, 3000, 2000]  Y_o=0  ydot_o=0  Izz=4000  psi_o=0  r_o=0  Af=2  Cd=.3  Cl=.1  Cpm=.1  beta_w=[0 0.01:0.01:0.3]  Cs=[0:0.03:0.9]  Cym=[0 1e-6:0.01:0.3]  Pabs=101325  Tair=273  g=9.81  mu=1  xdot_tol=.01  Fznom=5000  Fxtire_sat=7e4  Fytire_sat=7e4  longOff=0  latOff=0  vertOff=0  wrapAng=off
      settings: LibrarySourceBlock=vehdynlibeom/Vehicle Body 3DOF Dual Track
  XY Graph{1..6} (6 alike) : Record  Commented=on  NumPorts=2.0  FileSettingsInternal="{\"entries\":[{\"content\":{\"excelSettings\":{\"content\":{},\"type\":\"Streamout.ExcelSettings\"},\"parquetSettings\":{\"content\":{},\"type\":\"Streamout.ParquetSettings\"}},\"type\":\"Streamout.FileSettingStorage\",\"uuid\":\"\"}],\"packageUris\":[\"http:\\/\\/schema.mathworks.com\\/mf0\\/streamout_blocks\\/R2020a\"],\"version\":\"1.0\"}"  FrameSettings=[0, 0]  Layout=[1 1]  SignalsInternal="{\"entries\":[{\"content\":{},\"type\":\"RecordBlkView.InputSignals\",\"uuid\":\"\"}],\"packageUris\":[\"http:\\/\\/schema.mathworks.com\\/mf0\\/streamout_blocks\\/R2020a\"],\"version\":\"1.0\"}"  VisualizationBindings="{\"xyplotplugin\":{\"info\":[{\"series\":[],\"subplotID\":1}]}}"  CompatibilityTag=XY
  lf : Constant  Commented=on  Value=1.4
  lr : Constant  Commented=on  Value=1.6
  x_feedback1 : From  Commented=on  GotoTag=x_feedback
  x_feedback2 : From  Commented=on  GotoTag=x_feedback
  x_feedback4 : From  Commented=on  GotoTag=x_feedback
  x_feedback5 : From  Commented=on  GotoTag=x_feedback2
  y_feedback1 : From  Commented=on  GotoTag=y_feedback
  y_feedback2 : From  Commented=on  GotoTag=y_feedback
  y_feedback4 : From  Commented=on  GotoTag=y_feedback
  y_feedback5 : From  Commented=on  GotoTag=y_feedback2
  wires:
  Bicycle Kinematic Model/2 -> Demux1/1
  Bicycle Kinematic Model/1 -> Demux/1
  Demux/1 -> Goto5/1, XY Graph3/1  "x"
  Demux/2 -> Goto6/1, XY Graph3/2  "y"
  Demux/3 -> Display/1  "yaw"
  Demux1/1 -> Integrator/1, Scope/1  "x_dot"
  Demux1/2 -> Integrator1/1, Scope/2  "y_dot"
  Demux1/3 -> Integrator2/1, Scope/3  "w"
  Integrator2/1 -> Display1/1
  Integrator/1 -> XY Graph4/1  "x"
  Integrator1/1 -> XY Graph4/2  "y"
  Linear Velocity/1 -> Goto/1
  From/1 -> Bicycle Kinematic Model/1
  From1/1 -> Bicycle Kinematic Model/2
  lr/1 -> Add/1
  lf/1 -> Add/2
  Add/1 -> Goto3/1  "wheel base"
  From3/1 -> Tan/1
  Tan/1 -> Product/1
  From2/1 -> Product/2
  Product/1 -> Divide/1
  From4/1 -> Divide/2
  Divide/1 -> Integrator3/1
  Integrator3/1 -> Display2/1, Cos/1, Sin/1  "yaw"
  Cos/1 -> Product1/1
  Sin/1 -> Product2/2
  From5/1 -> Product2/1, Product1/2
  Product1/1 -> Integrator4/1
  Product2/1 -> Integrator5/1
  Integrator4/1 -> Goto2/1, XY Graph2/1  "x"
  Integrator5/1 -> XY Graph2/2, Goto4/1  "y"
  From6/1 -> Vehicle Body 3DOF Single Track1/1
  From7/1 -> Vehicle Body 3DOF Single Track1/2
  Vehicle Body 3DOF Single Track1/7 -> Terminator1/1
  From8/1 -> Ackermann Kinematic Model/1
  From9/1 -> Scope9/2, Derivative/1
  Derivative/1 -> Scope9/1, Ackermann Kinematic Model/2
  Ackermann Kinematic Model/1 -> Demux2/1
  Demux2/1 -> XY Graph5/1, Goto7/1  "x"
  Demux2/2 -> Goto8/1, XY Graph5/2  "y"
  Demux2/3 -> Display4/1  "q"
  Ackermann Kinematic Model/2 -> Terminator3/1
  Demux2/4 -> Display5/1  "steering angle"
  Angular Velocity/1 -> Scope3/1, Goto1/1
  From10/1 -> Scope1/1  "bicycle_block_x"
  From11/1 -> Scope1/2  "bicycle_block_y"
  From12/1 -> Scope1/3  "bicycle_sub_x"
  From13/1 -> Scope1/4  "bicycle_sub_y"
  From14/1 -> Scope1/5  "ackerman_block_x"
  From15/1 -> Scope1/6  "ackerman_block_y"
  From16/1 -> Scope1/7  "bicycle_vel_x"
  From17/1 -> Scope1/8  "bicycle_vel_y"
  From18/1 -> Scope2/1  "bicycle_block_x"
  From19/1 -> Scope2/2  "bicycle_block_y"
  From20/1 -> Scope2/3  "ackerman_block_x"
  From21/1 -> Scope2/4  "ackerman_block_y"
  From25/1 -> Scope4/4  "ackerman_block_y"
  From22/1 -> Scope4/1  "bicycle_block_x"
  From23/1 -> Scope4/2  "bicycle_block_y"
  From24/1 -> Scope4/3  "ackerman_block_x"
  From43/1 -> Product9/1
  From44/1 -> Cos1/1
  Cos1/1 -> Product9/2
  Cos2/1 -> Product10/2
  From45/1 -> Product10/1
  From46/1 -> Cos2/1
  Product9/1 -> Goto20/1, Integrator8/1
  Product10/1 -> Goto21/1, Integrator10/1
  Integrator8/1 -> XY Graph6/1, Goto14/1
  Integrator10/1 -> XY Graph6/2, Goto15/1
  From26/1 -> Scope5/1  "custom ackermann x"
  From30/1 -> Scope5/2  "custom ackermann y"
  From31/1 -> Scope5/3  "built-in ackermann x"
  From32/1 -> Scope5/4  "built-in ackermann y"
  From34/1 -> Scope6/2  "custom ackermann y"
  From33/1 -> Scope6/1  "custom ackermann x"
  From36/1 -> Scope6/4  "custom bicycle y"
  From35/1 -> Scope6/3  "custom bicycle x"
  Constant/1 -> Goto11/1
  From38/1 -> Tan2/1
  Tan2/1 -> Divide2/2
  Divide2/1 -> Goto16/1
  From39/1 -> Divide2/1
  From40/1 -> Gain1/1, Gain/1
  Gain/1 -> Add1/1
  From41/1 -> Add2/1, Add1/2
  Gain1/1 -> Add2/2
  From37/1 -> Divide3/1
  From42/1 -> Divide3/2
  Divide3/1 -> Goto17/1, Integrator11/1, Display8/1
  Add1/1 -> Product4/1
  From47/1 -> Product5/1, Product4/2
  Add2/1 -> Product5/2
  Product4/1 -> Goto18/1
  Product5/1 -> Goto19/1
  From48/1 -> Tan3/1
  Tan3/1 -> Product7/1, Product6/1
  From49/1 -> Add3/1, Product6/2
  Product6/1 -> Divide4/1
  From50/1 -> Gain2/1
  Gain2/1 -> Product7/2
  Product7/1 -> Add3/2
  Add3/1 -> Divide4/2
  Divide4/1 -> Goto22/1
  Product11/1 -> Add4/2
  From51/1 -> Tan4/1
  Product8/1 -> Divide5/1
  From52/1 -> Add4/1, Product8/2
  Divide5/1 -> Goto23/1
  Gain3/1 -> Product11/2
  Add4/1 -> Divide5/2
  From53/1 -> Gain3/1
  Tan4/1 -> Product11/1, Product8/1
  From54/1 -> Add5/1
  From55/1 -> Add5/2
  Add5/1 -> Gain4/1
  Gain4/1 -> Scope7/1  "feedback"
  From56/1 -> Scope7/2  "calculation"
  From58/1 -> Scope8/1  "Inner"
  From57/1 -> Scope8/2  "Steerıng Command"
  From59/1 -> Scope8/3  "Outer Wheel"
  Integrator11/1 -> Goto24/1
  Constant2/1 -> Vehicle Body 3DOF Single Track/3
  Constant3/1 -> Vehicle Body 3DOF Single Track/4
  Constant4/1 -> Vehicle Body 3DOF Single Track/5
  Constant7/1 -> Pure Pursuit/3
  Constant8/1 -> Pure Pursuit/4
  Constant5/1 -> Matrix Concatenate/1
  Constant6/1 -> Matrix Concatenate/2
  Matrix Concatenate/1 -> Pure Pursuit/2, Selector/1
  Vehicle Body 3DOF Single Track/1 -> Bus Selector/1
  Bus Selector/1 -> Goto25/1, Mux/1  "<X>"
  Bus Selector/2 -> Goto26/1, Mux/2  "<Y>"
  Bus Selector/3 -> Mux/3  "<psi>"
  Mux/1 -> Pure Pursuit/1
  Pure Pursuit/2 -> Terminator4/1
  Constant10/1 -> Product3/1
  Constant9/1 -> Product3/2
  Product3/1 -> Product12/1
  Sine Wave/1 -> Product12/2
  Pure Pursuit/3 -> Sine Wave/1
  Product12/1 -> Divide1/1
  Constant11/1 -> Divide1/2
  Divide1/1 -> Atan/1
  Vehicle Body 3DOF Single Track/7 -> Terminator5/1
  Vehicle Body 3DOF Single Track/6 -> Terminator6/1
  Vehicle Body 3DOF Single Track/5 -> Terminator7/1
  Vehicle Body 3DOF Single Track/4 -> Terminator8/1
  Vehicle Body 3DOF Single Track/3 -> Terminator9/1
  Vehicle Body 3DOF Single Track/2 -> Terminator10/1
  Selector/1 -> Demux3/1
  Demux3/1 -> Add6/1
  Demux3/2 -> Add7/1
  From27/1 -> Add6/2
  From28/1 -> Add7/2
  Add6/1 -> Dot Product/1, Dot Product/2
  Add7/1 -> Dot Product1/1, Dot Product1/2
  Dot Product/1 -> Add8/1
  Dot Product1/1 -> Add8/2
  Constant12/1 -> Less Than/2
  Add8/1 -> Square/1
  Square/1 -> Less Than/1
  Clock/1 -> Display6/1
  Pure Pursuit/1 -> Goto12/1
  Mux1/1 -> To Workspace/1
  x_feedback1/1 -> To Workspace1/1, Mux1/1
  y_feedback1/1 -> To Workspace2/1, Mux1/2
  Vehicle Body 3DOF Single Track1/6 -> Terminator11/1
  Vehicle Body 3DOF Single Track1/5 -> Terminator12/1
  Vehicle Body 3DOF Single Track1/4 -> Display3/1
  Vehicle Body 3DOF Single Track1/3 -> Terminator13/1
  Vehicle Body 3DOF Single Track1/2 -> Terminator14/1
  Vehicle Body 3DOF Single Track1/1 -> Bus Selector1/1
  Bus Selector1/1 -> XY Graph1/1, Goto9/1  "<X>"
  Bus Selector1/2 -> XY Graph1/2, Goto10/1  "<Y>"
  From29/1 -> Vehicle Body 3DOF Single Track/2
  Less Than/1 -> Stop Simulation/1
  Subscribe/2 -> Bus Selector4/1, To Workspace3/1
  Subscribe/1 -> Scope10/1
  Atan/1 -> Goto13/1
  From60/1 -> Vehicle Body 3DOF Single Track/1
  Vehicle Body 3DOF Single Track2/6 -> Terminator17/1
  Atan1/1 -> Goto28/1
  Divide6/1 -> Atan1/1
  Add9/1 -> Dot Product2/1, Dot Product2/2
  Demux4/1 -> Add9/1
  Pure Pursuit1/2 -> Terminator15/1
  Matrix Concatenate1/1 -> Pure Pursuit1/2, Selector1/1
  Vehicle Body 3DOF Single Track2/7 -> Terminator16/1
  Product13/1 -> Divide6/1
  Less Than1/1 -> Stop Simulation1/1
  Constant16/1 -> Vehicle Body 3DOF Single Track2/4
  Constant18/1 -> Matrix Concatenate1/1
  Add10/1 -> Dot Product3/1, Dot Product3/2
  Vehicle Body 3DOF Single Track2/2 -> Terminator2/1
  Bus Selector2/1 -> Goto29/1, Mux2/1  "<X>"
  Bus Selector2/3 -> Mux2/3  "<psi>"
  Constant17/1 -> Vehicle Body 3DOF Single Track2/5
  Constant15/1 -> Vehicle Body 3DOF Single Track2/3
  From63/1 -> Vehicle Body 3DOF Single Track2/2
  Vehicle Body 3DOF Single Track2/1 -> Bus Selector2/1
  Dot Product2/1 -> Add11/1
  Constant13/1 -> Divide6/2
  Clock1/1 -> Display7/1
  Vehicle Body 3DOF Single Track2/4 -> Terminator19/1
  From64/1 -> Vehicle Body 3DOF Single Track2/1, Scope17/1
  y_feedback2/1 -> To Workspace6/1, Mux3/2
  x_feedback2/1 -> To Workspace5/1, Mux3/1
  From62/1 -> Add10/2
  Constant19/1 -> Matrix Concatenate1/2
  Constant14/1 -> Less Than1/2
  Add11/1 -> Square1/1
  From61/1 -> Add9/2
  Demux4/2 -> Add10/1
  Sine Wave1/1 -> Product13/2
  Dot Product3/1 -> Add11/2
  Mux3/1 -> To Workspace4/1
  Vehicle Body 3DOF Single Track2/5 -> Terminator18/1
  Constant22/1 -> Product14/2
  Bus Selector2/2 -> Goto30/1, Mux2/2  "<Y>"
  Constant1/1 -> Product14/1
  Vehicle Body 3DOF Single Track2/3 -> Terminator20/1
  Square1/1 -> Less Than1/1
  Mux2/1 -> Pure Pursuit1/1
  Selector1/1 -> Demux4/1
  Product14/1 -> Product13/1
  Pure Pursuit1/1 -> Scope13/1, Goto27/1
  Constant23/1 -> Add12/2, Add13/1
  Constant24/1 -> Add13/2
  Add12/1 -> Divide7/1
  Add13/1 -> Divide7/2
  Constant26/1 -> Add15/2, Add14/2
  Constant25/1 -> Add14/1
  Divide7/1 -> Product15/1
  Add14/1 -> Product15/2
  Product15/1 -> Add15/1
  Constant21/1 -> Manual Switch/1
  Manual Switch/1 -> Pure Pursuit1/4
  From66/1 -> Manual Switch/2
  Constant31/1 -> Add19/2, Add18/1
  Constant30/1 -> Add17/2
  Add17/1 -> Divide8/2
  From67/1 -> Add16/1
  Constant29/1 -> Add17/1, Add16/2
  Product16/1 -> Add19/1
  Add18/1 -> Product16/2
  Constant32/1 -> Add18/2
  Divide8/1 -> Product16/1
  Add16/1 -> Divide8/1
  Constant20/1 -> Manual Switch1/1
  From68/1 -> Manual Switch1/2
  From69/1 -> Scope11/2  "steer_cmd"
  From65/1 -> Abs/1
  Abs/1 -> Add12/1
  From70/1 -> Scope12/2  "steer_cmd"
  Pure Pursuit1/3 -> Sine Wave1/1
  From77/1 -> Scope19/1  "reg_ld"
  From78/1 -> Scope19/2  "reg_vel"
  Add19/1 -> Abs3/1  "regulated_vel"
  Abs3/1 -> Scope12/1, Goto32/1  "regulated_vel"
  Add15/1 -> Abs4/1  "regulated_ld"
  Abs4/1 -> Saturation/1, Scope11/1  "regulated_ld"
  Bus Selector4/1 -> To Workspace10/1  "<points>"
  Product23/1 -> Divide13/1
  From83/1 -> Add28/1
  Clock3/1 -> Display10/1
  Divide10/1 -> Atan3/1
  Add32/1 -> Abs2/1  "regulated_vel"
  Bus Selector5/1 -> Goto39/1, Mux6/1  "<X>"
  Divide12/1 -> Product22/1
  Vehicle Body 3DOF Single Track5/2 -> Terminator40/1
  Add26/1 -> Product21/2
  Bus Selector5/2 -> Goto40/1, Mux6/2  "<Y>"
  Bus Selector6/2 -> Goto46/1, Mux8/2  "<Y>"
  From82/1 -> Manual Switch2/2
  Add22/1 -> Dot Product7/1, Dot Product7/2
  Matrix Concatenate4/1 -> Pure Pursuit4/2, Selector4/1
  Constant61/1 -> Add32/2, Add31/1
  Demux6/1 -> Add36/1
  Add25/1 -> Divide11/2
  Dot Product7/1 -> Add23/2
  y_feedback5/1 -> To Workspace16/1, Mux9/2
  Constant56/1 -> Add27/2, Add26/2
  Sine Wave4/1 -> Product23/2
  Manual Switch3/1 -> Pure Pursuit3/3
  Matrix Concatenate3/1 -> Selector3/1, Pure Pursuit3/2
  Demux6/2 -> Add22/1
  Constant53/1 -> Add24/2, Add25/1
  Constant71/1 -> Product24/2
  Constant44/1 -> Less Than3/2
  Square4/1 -> Less Than4/1
  Add29/1 -> Divide12/2
  Mux8/1 -> Pure Pursuit4/1
  Vehicle Body 3DOF Single Track5/6 -> Terminator37/1
  Square3/1 -> Less Than3/1
  Constant46/1 -> Vehicle Body 3DOF Single Track4/4
  From84/1 -> Manual Switch3/2
  Mux6/1 -> Pure Pursuit3/1
  y_feedback4/1 -> To Workspace13/1, Mux7/2
  Constant62/1 -> Add31/2
  Divide13/1 -> Atan4/1
  Clock4/1 -> Display11/1
  Sine Wave3/1 -> Product19/2
  Constant43/1 -> Divide10/2
  Vehicle Body 3DOF Single Track4/2 -> Terminator33/1
  From76/1 -> Add22/2
  From92/1 -> Scope24/2  "reg_vel"
  Vehicle Body 3DOF Single Track5/7 -> Terminator36/1
  From75/1 -> Add36/2
  Constant65/1 -> Vehicle Body 3DOF Single Track5/4
  Add31/1 -> Product22/2
  From79/1 -> Vehicle Body 3DOF Single Track4/2
  Pure Pursuit3/3 -> Sine Wave3/1
  Demux7/2 -> Add33/1
  Add35/1 -> Dot Product8/1, Dot Product8/2
  Dot Product8/1 -> Add34/1
  Abs1/1 -> Add24/1
  Demux7/1 -> Add35/1
  Vehicle Body 3DOF Single Track4/5 -> Terminator31/1
  Abs5/1 -> Scope14/1, Goto41/1
  Pure Pursuit3/2 -> Terminator28/1
  Dot Product9/1 -> Add34/2
  Constant42/1 -> Product20/1
  Add27/1 -> Abs5/1  "regulated_ld"
  Constant47/1 -> Vehicle Body 3DOF Single Track4/5
  Product24/1 -> Product23/1
  Constant66/1 -> Vehicle Body 3DOF Single Track5/5
  Constant69/1 -> Pure Pursuit4/3
  From88/1 -> Add33/2
  Constant57/1 -> Product24/1
  Product19/1 -> Divide10/1
  Product21/1 -> Add27/1
  Dot Product6/1 -> Add23/1
  Mux7/1 -> To Workspace11/1
  Vehicle Body 3DOF Single Track5/4 -> Terminator39/1
  Add24/1 -> Divide11/1
  Constant52/1 -> Product20/2
  Pure Pursuit4/3 -> Sine Wave4/1
  Add34/1 -> Square4/1
  Divide11/1 -> Product21/1
  Abs2/1 -> Scope15/1, Goto42/1
  Atan4/1 -> Goto44/1
  From81/1 -> Abs1/1
  Constant59/1 -> Add29/1, Add28/2
  From91/1 -> Scope24/1  "reg_ld"
  Vehicle Body 3DOF Single Track4/6 -> Terminator30/1
  Vehicle Body 3DOF Single Track5/5 -> Terminator38/1
  From87/1 -> Add35/2
  From85/1 -> Scope14/2  "steer_cmd"
  Constant63/1 -> Less Than4/2
  Add36/1 -> Dot Product6/1, Dot Product6/2
  Manual Switch2/1 -> Pure Pursuit3/4
  Vehicle Body 3DOF Single Track4/3 -> Terminator34/1
  Constant70/1 -> Pure Pursuit4/4
  Less Than3/1 -> Stop Simulation3/1
  From80/1 -> Vehicle Body 3DOF Single Track4/1, Scope22/1
  Constant50/1 -> Manual Switch3/1
  Atan3/1 -> Goto38/1
  Constant45/1 -> Vehicle Body 3DOF Single Track4/3
  From89/1 -> Vehicle Body 3DOF Single Track5/2
  Pure Pursuit3/1 -> Scope20/1, Goto37/1
  Selector4/1 -> Demux7/1
  Vehicle Body 3DOF Single Track5/3 -> Terminator41/1
  Mux9/1 -> To Workspace14/1
  Bus Selector6/3 -> Mux8/3  "<psi>"
  x_feedback4/1 -> To Workspace12/1, Mux7/1
  Selector3/1 -> Demux6/1
  Constant58/1 -> Divide13/2
  x_feedback5/1 -> To Workspace15/1, Mux9/1
  Add23/1 -> Square3/1
  Constant54/1 -> Add25/2
  From86/1 -> Scope15/2  "steer_cmd"
  Vehicle Body 3DOF Single Track4/7 -> Terminator29/1
  Constant64/1 -> Vehicle Body 3DOF Single Track5/3
  Add33/1 -> Dot Product9/1, Dot Product9/2
  Constant55/1 -> Add26/1
  From90/1 -> Vehicle Body 3DOF Single Track5/1, Scope23/1
  Vehicle Body 3DOF Single Track4/1 -> Bus Selector5/1
  Vehicle Body 3DOF Single Track5/1 -> Bus Selector6/1
  Constant51/1 -> Manual Switch2/1
  Less Than4/1 -> Stop Simulation4/1
  Bus Selector5/3 -> Mux6/3  "<psi>"
  Constant60/1 -> Add29/2
  Pure Pursuit4/2 -> Terminator35/1
  Product22/1 -> Add32/1
  Vehicle Body 3DOF Single Track4/4 -> Terminator32/1
  Bus Selector6/1 -> Goto45/1, Mux8/1  "<X>"
  Add28/1 -> Divide12/1
  Product20/1 -> Product19/1
  Pure Pursuit4/1 -> Scope21/1, Goto43/1
  From95/1 -> Matrix Concatenate4/1
  From96/1 -> Matrix Concatenate4/2
  Constant48/1 -> Goto47/1
  Constant49/1 -> Goto48/1
  From93/1 -> Matrix Concatenate3/1
  From94/1 -> Matrix Concatenate3/2
  Manual Switch1/1 -> Pure Pursuit1/3
  Saturation/1 -> Goto31/1
  [steering_cmd] -> To Workspace17/1
  [regulated_vel] -> To Workspace18/1
  [regulated_ld] -> To Workspace19/1
  [x_feedback_nn] -> To Workspace21/1, Mux11/1
  Bus Selector7/1 -> [x_feedback_nn], Mux10/1  "<X>"
  Constant74/1 -> Vehicle Body 3DOF Single Track6/4
  Divide14/1 -> Atan5/1
  Mux10/1 -> Pure Pursuit5/1
  Vehicle Body 3DOF Single Track6/3 -> Terminator48/1
  Dot Product11/1 -> Add38/2
  Demux8/2 -> Add37/1
  Constant73/1 -> Vehicle Body 3DOF Single Track6/3
  [calculated_lin_vel_nn] -> Vehicle Body 3DOF Single Track6/2
  Vehicle Body 3DOF Single Track6/1 -> Bus Selector7/1
  Square5/1 -> Less Than5/1
  MATLAB Function1/2(velocity) -> Unit Delay1/1
  [y_feedback_nn] -> To Workspace22/1, Mux11/2
  Bus Selector7/2 -> [y_feedback_nn], Mux10/2  "<Y>"
  Pure Pursuit5/2 -> Terminator42/1
  Constant67/1 -> Product26/1
  Demux8/1 -> Add39/1
  Vehicle Body 3DOF Single Track6/2 -> Terminator47/1
  Vehicle Body 3DOF Single Track6/6 -> Terminator44/1
  Less Than5/1 -> Stop Simulation5/1
  Constant80/1 -> Product26/2
  Pure Pursuit5/1 -> Scope25/1, [calculated_lin_vel_nn]
  MATLAB Function1/1(lookahead) -> Unit Delay/1
  [y_feedback_nn] -> Add37/2
  Vehicle Body 3DOF Single Track6/5 -> Terminator45/1
  Sine Wave5/1 -> Product25/2
  Atan5/1 -> [steering_cmd_nn]
  Constant76/1 -> Vector Concatenate/1, Matrix Concatenate5/1
  Clock5/1 -> Display12/1
  Constant68/1 -> Divide14/2
  Matrix Concatenate5/1 -> Pure Pursuit5/2, Selector5/1
  Add37/1 -> Dot Product11/1, Dot Product11/2
  Dot Product10/1 -> Add38/1
  Add39/1 -> Dot Product10/1, Dot Product10/2
  Add38/1 -> Square5/1
  Constant72/1 -> Less Than5/2
  Constant77/1 -> Vector Concatenate/2, Matrix Concatenate5/2
  Pure Pursuit5/3 -> Sine Wave5/1
  Mux11/1 -> To Workspace20/1
  Selector5/1 -> Demux8/1
  Product26/1 -> Product25/1
  Product25/1 -> Divide14/1
  Constant75/1 -> Vehicle Body 3DOF Single Track6/5
  [steering_cmd_nn] -> Vehicle Body 3DOF Single Track6/1, Scope26/1
  Vehicle Body 3DOF Single Track6/7 -> Terminator43/1
  Vehicle Body 3DOF Single Track6/4 -> Terminator46/1
  Bus Selector7/3 -> Mux10/3  "<psi>"
  [x_feedback_nn] -> Add39/2
  [steering_cmd_nn] -> Vector Concatenate/3
  Vector Concatenate/1 -> MATLAB Function/1(u)
  Constant78/1 -> MATLAB Function/2(x_mean)
  Constant79/1 -> MATLAB Function/3(x_std)
  MATLAB Function/1(x_scaled) -> ONNX Model Predict/1
  Constant81/1 -> MATLAB Function1/2(y_mean)
  Constant82/1 -> MATLAB Function1/3(y_std)
  ONNX Model Predict/1 -> MATLAB Function1/1(y_scaled)
  Unit Delay/1 -> Pure Pursuit5/3
  Unit Delay1/1 -> Pure Pursuit5/4

== matlab function pure_pursuit/MATLAB Function1 ==
  data: y_scaled input; lookahead output; y_mean input; y_std input; velocity output
function [lookahead, velocity] = denormalize_output(y_scaled, y_mean, y_std)

lookahead = double(y_scaled(1,1)) * double(y_std(1)) + double(y_mean(1));
velocity  = double(y_scaled(1,2)) * double(y_std(2)) + double(y_mean(2));

% Safety limits
lookahead = max(lookahead, 1.0);
velocity  = max(velocity, 0.0);

end

== matlab function pure_pursuit/MATLAB Function ==
  data: u input; x_scaled output; x_mean input; x_std input
function x_scaled = normalize_input(u, x_mean, x_std)

x_scaled = zeros(1,3,'single');

x_scaled(1,1) = single((u(1) - x_mean(1)) / x_std(1));
x_scaled(1,2) = single((u(2) - x_mean(2)) / x_std(2));
x_scaled(1,3) = single((u(3) - x_mean(3)) / x_std(3));

end
